simulink model "P8_DCMotor_simulink"  (R2023a)
settings: Solver=VariableStepAuto  StartTime=0.0  StopTime=10.0  RelTol=1e-3
values from neighbouring files (symbols this model uses):
  b = 1.2e-3    (= 0.0012)    [P8_DCMotor.m]
  J = 1e-3    (= 0.001)    [P8_DCMotor.m]
  Ke = 0.01    [P8_DCMotor.m]
  Kt = 0.01    [P8_DCMotor.m]
  La = 0.023    [P8_DCMotor.m]
  Ra = 2    [P8_DCMotor.m]
settings Model: Creator=karen  LastModifiedBy=karen

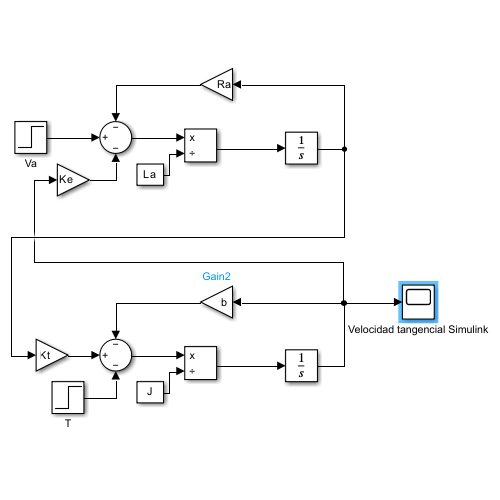
[thumbnail: Simulink's stored preview of the top-level diagram]
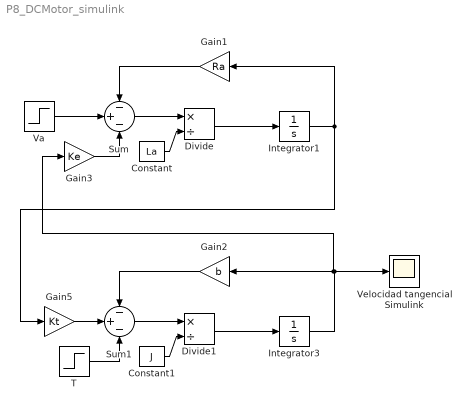
== system P8_DCMotor_simulink ==
  Constant : Constant  Value=La
  Constant1 : Constant  Value=J
  Divide : Product  Inputs=*/
  Divide1 : Product  Inputs=*/
  Gain1 : Gain  Gain=Ra
  Gain2 : Gain  Gain=b
  Gain3 : Gain  Gain=Ke
  Gain5 : Gain  Gain=Kt
  Integrator1 : Integrator
  Integrator3 : Integrator
  Sum : Sum  Inputs=-+-
  Sum1 : Sum  Inputs=-+-
  T : Step  Time=0  After=0  SampleTime=0
  Va : Step  Time=0  After=5  SampleTime=0
  Velocidad tangencial Simulink : Scope
  wires:
  Divide/1 -> Integrator1/1
  Gain3/1 -> Sum/3
  Sum/1 -> Divide/1
  Constant/1 -> Divide/2
  Va/1 -> Sum/2
  Gain1/1 -> Sum/1
  Integrator1/1 -> Gain1/1, Gain5/1
  Divide1/1 -> Integrator3/1
  Gain2/1 -> Sum1/1
  Constant1/1 -> Divide1/2
  Integrator3/1 -> Gain3/1, Gain2/1, Velocidad tangencial Simulink/1
  T/1 -> Sum1/3
  Sum1/1 -> Divide1/1
  Gain5/1 -> Sum1/2
